simulink model "master_Hinf_sampled_sys"  (R2015a)
settings: Solver=ode45  SolverMode=SingleTasking  StartTime=0.0  StopTime=10.0  RelTol=1e-3
values from neighbouring files (symbols this model uses):
  A = [0 1; 0 -Bm/Mm]    [master_Hinf.m]
  B = [0; 1/Mm]    [master_Hinf.m]
  C = [1 0; 0 1]    [master_Hinf.m]
  D = [0; 0]    [master_Hinf.m]
  K = M_s * Q_s'    [master_Hinf.m]
undefined symbols (not defined in the file or in its folder): Ad, Bd, Cd, Dd, Ts
settings Model: Creator=enrico-giordano  LastModifiedBy=enrico-giordano
settings OptimizationCC: BlockReduction=off  BooleanDataType=off
settings DebuggingCC: SaveWithParameterizedLinksMsg=none  UnderspecifiedInitializationDetection=Classic  MergeDetectMultiDrivingBlocksExec=none  SignalResolutionControl=TryResolveAllWithWarning
settings HardwareCC: TargetUnknown=on

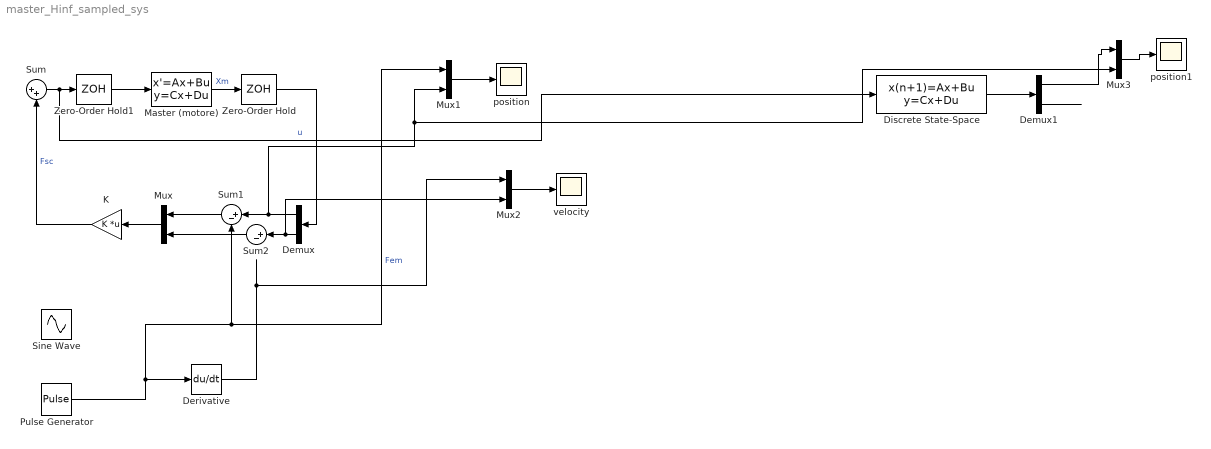
== system master_Hinf_sampled_sys ==
  Demux : Demux  Outputs=2
  Demux1 : Demux  Outputs=2
  Derivative : Derivative
  Discrete State-Space : DiscreteStateSpace  A=Ad  B=Bd  C=Cd  D=Dd  SampleTime=Ts
  K : Gain  Gain=K  Multiplication=Matrix(K*u)
  Master (motore) : StateSpace  A=A  B=B  C=C  D=D  X0=0
  Mux{,1..3} (4 alike) : Mux  Inputs=2
  Pulse Generator : DiscretePulseGenerator  PulseType=Time based  PulseWidth=50
  Sine Wave : Sin  Amplitude=10  SampleTime=0
  Sum : Sum  Inputs=|++
  Sum1 : Sum  Inputs=|+-
  Sum2 : Sum  Inputs=|+-
  Zero-Order Hold : ZeroOrderHold  SampleTime=Ts
  Zero-Order Hold1 : ZeroOrderHold  SampleTime=Ts
  position : Scope
      settings: TimeRange=10  YMin=-0.6000000000000001  YMax=0.2
  position1 : Scope
      settings: TimeRange=10  YMin=-0.6000000000000001  YMax=0.2  SaveName=ScopeData2
  velocity : Scope
      settings: TimeRange=10  YMin=-0.6000000000000001  YMax=0.2
  wires:
  Sum/1 -> Zero-Order Hold1/1, Discrete State-Space/1  "u"
  Master (motore)/1 -> Zero-Order Hold/1  "Xm"
  K/1 -> Sum/2  "Fsc"
  Mux/1 -> K/1
  Demux/1 -> Mux3/2, Mux1/2, Sum1/1
  Sum1/1 -> Mux/1
  Pulse Generator/1 -> Sum1/2, Mux1/1, Derivative/1  "Fem"
  Demux/2 -> Mux2/2, Sum2/1
  Mux1/1 -> position/1
  Sum2/1 -> Mux/2
  Derivative/1 -> Mux2/1
  Mux2/1 -> velocity/1
  Zero-Order Hold/1 -> Demux/1
  Zero-Order Hold1/1 -> Master (motore)/1
  Discrete State-Space/1 -> Demux1/1
  Demux1/1 -> Mux3/1
  Mux3/1 -> position1/1
  Demux1/2 -> ?
